simulink model "snb_d"  (R2012b)
settings: Solver=FixedStepDiscrete  SolverMode=SingleTasking  StartTime=0.0  StopTime=10000  RelTol=1e-3
undefined symbols (not defined in the file): Down, pfb_coeff_gen_calc, Up, xlipgetpartsetting
libraries: xbsIndex_r4 x12106, casper_library_misc x14, casper_library_communications x8, casper_library_delays x1, xps_library x1
(part 24 of 79)

== system snb_d/mix_dec_fir/dec_fir_async1 ==
  sync_in : Inport
  dv_in : Inport  Port=2
  dbus_in : Inport  Port=3
  convert1 : xbsIndex_r4/Convert  gui_display_data_type=Fixed-point  arith_type="Signed  (2's comp)"  n_bits=18  bin_pt=17  float_type=Single  exp_bits=8  fraction_bits=24  quantization="Round  (unbiased: +/- Inf)"  overflow=Wrap  en=off  latency=3  dbl_ovrd=off  pipeline=off  block_type=convert
  convert2 : xbsIndex_r4/Convert  gui_display_data_type=Fixed-point  arith_type="Signed  (2's comp)"  n_bits=18  bin_pt=17  float_type=Single  exp_bits=8  fraction_bits=24  quantization="Round  (unbiased: +/- Inf)"  overflow=Wrap  en=off  latency=3  dbl_ovrd=off  pipeline=off  block_type=convert
  dv_delay : xbsIndex_r4/Delay  rst=off  infoeditControl=Selection of Reset will increase slice count due to use of real FFs and instead of SRLs  en=off  latency=18  dbl_ovrd=off  reg_retiming=off  block_type=delay
  fir_col_async1 : Subsystem  AncestorBlock=casper_library_downconverter/fir_col_async  mask(fir_col_async){n_inputs=8, coeff=[0.12401     0.11348    0.094703    0.071556    0.048306    0.028458    0.013979   0.0055083], add_latency=3, mult_latency=3, coeff_bit_width=24, coeff_bin_pt=23, first_stage_hdl=on, adder_imp=DSP48, async=on, bus_input=on, input_width=20, input_bp=18, input_type=Signed, dbl=on}
      mask prompts: n_inputs "Inputs"; coeff "Coefficients"; add_latency "Add latency"; mult_latency "Mult Latency"; coeff_bit_width "Coefficient bit width"; coeff_bin_pt "Coefficient binary point"; first_stage_hdl "Implement first stage of adder trees on output as behavioural HDL"; adder_imp "Adder implementation"; async "Asynchronous ops"; bus_input "Bus input"; input_width "Input bitwidth"; input_bp "Input binary point"; input_type "Input datatype"; dbl "Double col"
      mask init:
      | fir_col_async_init(gcb);
      mask Help: eval('xlWeb(''http://casper.berkeley.edu/wiki/Fir_col'')')
      mask TypeOptions adder_imp: Behavioral | Fabric | DSP48
      mask Callback bus_input:
      | onoff = get_param(gcb, 'bus_input');
      | set_param_state(gcb, 'input_width', onoff)
      | set_param_state(gcb, 'input_bp', onoff)
      | set_param_state(gcb, 'input_type', onoff)
      mask TypeOptions input_type: Signed | Unsigned
  imag_sum : Subsystem  AncestorBlock=casper_library_misc/adder_tree  mask(adder_tree){n_inputs=1, latency=3, adder_imp=DSP48, first_stage_hdl=off}
      mask prompts: n_inputs "Number of Inputs"; latency "Add Latency"; adder_imp "Adder implementation"; first_stage_hdl "Use behavioural HDL for first stage of adders"
      mask help:
      | Sums all inputs using a tree of adds and delays.
      |
      | Number of inputs: The number of inputs to the block to be summed
      | Add latency: The number of clock cycles to perform one addition (affects timing)..
      | Adder implementation: choice of fabric or DSP48E core, or behavioral HDL
      | Use behavioural HDL for first stage of adders: Causes the first stage of adders to be absorbed into DSP blocks if multipliers precede them (Virtex 5). Overrides Adder implementation
      mask init:
      | adder_tree_init(gcb, ...
      |     'n_inputs', n_inputs, ...
      |     'latency', latency, ...
      |     'adder_imp', adder_imp, ...
      |     'first_stage_hdl', first_stage_hdl);
      settings: AttributesFormatString=latency 0
      mask Help: eval('xlWeb(''http://casper.berkeley.edu/wiki/Adder_tree'')')
      mask TypeOptions adder_imp: Behavioral | Fabric | DSP48
  real_sum : Subsystem  AncestorBlock=casper_library_misc/adder_tree  mask(adder_tree){n_inputs=1, latency=3, adder_imp=DSP48, first_stage_hdl=off}
      mask prompts: n_inputs "Number of Inputs"; latency "Add Latency"; adder_imp "Adder implementation"; first_stage_hdl "Use behavioural HDL for first stage of adders"
      mask help:
      | Sums all inputs using a tree of adds and delays.
      |
      | Number of inputs: The number of inputs to the block to be summed
      | Add latency: The number of clock cycles to perform one addition (affects timing)..
      | Adder implementation: choice of fabric or DSP48E core, or behavioral HDL
      | Use behavioural HDL for first stage of adders: Causes the first stage of adders to be absorbed into DSP blocks if multipliers precede them (Virtex 5). Overrides Adder implementation
      mask init:
      | adder_tree_init(gcb, ...
      |     'n_inputs', n_inputs, ...
      |     'latency', latency, ...
      |     'adder_imp', adder_imp, ...
      |     'first_stage_hdl', first_stage_hdl);
      settings: AttributesFormatString=latency 0
      mask Help: eval('xlWeb(''http://casper.berkeley.edu/wiki/Adder_tree'')')
      mask TypeOptions adder_imp: Behavioral | Fabric | DSP48
  ri_to_c : casper_library_misc/ri_to_c
  shift1 : xbsIndex_r4/Shift  shift_dir=Left  shift_bits=0  en=off  latency=0  precision=Full  arith_type="Signed  (2's comp)"  n_bits=16  bin_pt=14  quantization=Truncate  overflow=Wrap  dbl_ovrd=off  block_type=shift
  shift2 : xbsIndex_r4/Shift  shift_dir=Left  shift_bits=0  en=off  latency=0  precision=Full  arith_type="Signed  (2's comp)"  n_bits=16  bin_pt=14  quantization=Truncate  overflow=Wrap  dbl_ovrd=off  block_type=shift
  sync_delay : xbsIndex_r4/Delay  rst=off  infoeditControl=Selection of Reset will increase slice count due to use of real FFs and instead of SRLs  en=off  latency=18  dbl_ovrd=off  reg_retiming=off  block_type=delay
  sync_out : Outport
  dout : Outport  Port=2
  dv_out : Outport  Port=3
  wires:
  sync_in/1 -> sync_delay/1
  dv_in/1 -> dv_delay/1, fir_col_async1/3(dv)
  dv_delay/1 -> dv_out/1
  dbus_in/1 -> fir_col_async1/1(dbus_in)
  fir_col_async1/3(real_sum) -> real_sum/2(din1)
  fir_col_async1/4(imag_sum) -> imag_sum/2(din1)
  real_sum/2(dout) -> shift1/1
  imag_sum/2(dout) -> shift2/1
  shift1/1 -> convert1/1
  shift2/1 -> convert2/1
  convert1/1 -> ri_to_c/1
  convert2/1 -> ri_to_c/2
  ri_to_c/1 -> dout/1
  sync_delay/1 -> real_sum/1(sync), imag_sum/1(sync)
  real_sum/1(sync_out) -> sync_out/1
  fir_col_async1/1(dbus_out) -> fir_col_async1/2(dbus_back_in)

== system snb_d/mix_dec_fir/mixer ==
  sync : Inport
  din1 : Inport  Port=2
  din2 : Inport  Port=3
  din3 : Inport  Port=4
  din4 : Inport  Port=5
  din5 : Inport  Port=6
  din6 : Inport  Port=7
  din7 : Inport  Port=8
  din8 : Inport  Port=9
  dds : Subsystem  AncestorBlock=casper_library_downconverter/dds  mask(dds){freq_div=16, freq=4, num_lo=8, n_bits=10, latency=2}
      mask prompts: freq_div "Frequency divisions (M)"; freq "Frequency (? / M*2pi)"; num_lo "Parallel LOs"; n_bits "Bit Width"
      mask help:
      | Generates P channels of sin and cos data for mixing
      | with input data in a DDC. To generate frequency
      | N/M(Fc x P) (where Fc is the clock rate)
      | M = "Frequency Divisions", N = "Frequency",
      | Parallel LOs = P
      mask init:
      | dds_init(gcb, ...
      |     'freq_div', freq_div, ...
      |     'freq', freq, ...
      |     'num_lo', num_lo, ...
      |     'n_bits', n_bits, ...
      |     'latency', latency);
      settings: AttributesFormatString=lo at -4/16
      mask Help: eval('xlWeb(''http://casper.berkeley.edu/wiki/Dds'')')
  delay : xbsIndex_r4/Delay  rst=off  infoeditControl=Selection of Reset will increase slice count due to use of real FFs and instead of SRLs  en=off  latency=4  dbl_ovrd=off  reg_retiming=off  block_type=delay
  rcmult1 : Subsystem  AncestorBlock=casper_library_downconverter/rcmult  mask(rcmult){latency=4}
      mask prompts: latency "Multiplier latency"
      mask help:
      | Multiplies input data with cos and sin inputs and
      | outputs results on real and imag ports
      | respectively.
      mask init:
      | rcmult_init(gcb, ...
      |     'latency', latency);
      mask Help: eval('xlWeb(''http://casper.berkeley.edu/wiki/Rcmult'')')
  rcmult2 : Subsystem  AncestorBlock=casper_library_downconverter/rcmult  mask(rcmult){latency=4}
      mask prompts: latency "Multiplier latency"
      mask help:
      | Multiplies input data with cos and sin inputs and
      | outputs results on real and imag ports
      | respectively.
      mask init:
      | rcmult_init(gcb, ...
      |     'latency', latency);
      mask Help: eval('xlWeb(''http://casper.berkeley.edu/wiki/Rcmult'')')
  rcmult3 : Subsystem  AncestorBlock=casper_library_downconverter/rcmult  mask(rcmult){latency=4}
      mask prompts: latency "Multiplier latency"
      mask help:
      | Multiplies input data with cos and sin inputs and
      | outputs results on real and imag ports
      | respectively.
      mask init:
      | rcmult_init(gcb, ...
      |     'latency', latency);
      mask Help: eval('xlWeb(''http://casper.berkeley.edu/wiki/Rcmult'')')
  rcmult4 : Subsystem  AncestorBlock=casper_library_downconverter/rcmult  mask(rcmult){latency=4}
      mask prompts: latency "Multiplier latency"
      mask help:
      | Multiplies input data with cos and sin inputs and
      | outputs results on real and imag ports
      | respectively.
      mask init:
      | rcmult_init(gcb, ...
      |     'latency', latency);
      mask Help: eval('xlWeb(''http://casper.berkeley.edu/wiki/Rcmult'')')
  rcmult5 : Subsystem  AncestorBlock=casper_library_downconverter/rcmult  mask(rcmult){latency=4}
      mask prompts: latency "Multiplier latency"
      mask help:
      | Multiplies input data with cos and sin inputs and
      | outputs results on real and imag ports
      | respectively.
      mask init:
      | rcmult_init(gcb, ...
      |     'latency', latency);
      mask Help: eval('xlWeb(''http://casper.berkeley.edu/wiki/Rcmult'')')
  rcmult6 : Subsystem  AncestorBlock=casper_library_downconverter/rcmult  mask(rcmult){latency=4}
      mask prompts: latency "Multiplier latency"
      mask help:
      | Multiplies input data with cos and sin inputs and
      | outputs results on real and imag ports
      | respectively.
      mask init:
      | rcmult_init(gcb, ...
      |     'latency', latency);
      mask Help: eval('xlWeb(''http://casper.berkeley.edu/wiki/Rcmult'')')
  rcmult7 : Subsystem  AncestorBlock=casper_library_downconverter/rcmult  mask(rcmult){latency=4}
      mask prompts: latency "Multiplier latency"
      mask help:
      | Multiplies input data with cos and sin inputs and
      | outputs results on real and imag ports
      | respectively.
      mask init:
      | rcmult_init(gcb, ...
      |     'latency', latency);
      mask Help: eval('xlWeb(''http://casper.berkeley.edu/wiki/Rcmult'')')
  rcmult8 : Subsystem  AncestorBlock=casper_library_downconverter/rcmult  mask(rcmult){latency=4}
      mask prompts: latency "Multiplier latency"
      mask help:
      | Multiplies input data with cos and sin inputs and
      | outputs results on real and imag ports
      | respectively.
      mask init:
      | rcmult_init(gcb, ...
      |     'latency', latency);
      mask Help: eval('xlWeb(''http://casper.berkeley.edu/wiki/Rcmult'')')
  sync_out : Outport
  real1 : Outport  Port=2
  imag1 : Outport  Port=3
  real2 : Outport  Port=4
  imag2 : Outport  Port=5
  real3 : Outport  Port=6
  imag3 : Outport  Port=7
  real4 : Outport  Port=8
  imag4 : Outport  Port=9
  real5 : Outport  Port=10
  imag5 : Outport  Port=11
  real6 : Outport  Port=12
  imag6 : Outport  Port=13
  real7 : Outport  Port=14
  imag7 : Outport  Port=15
  real8 : Outport  Port=16
  imag8 : Outport  Port=17
  wires:
  sync/1 -> delay/1
  delay/1 -> sync_out/1
  din1/1 -> rcmult1/1(d)
  dds/1(sin0) -> rcmult1/2(sin)
  dds/2(cos0) -> rcmult1/3(cos)
  rcmult1/1(real) -> real1/1
  rcmult1/2(imag) -> imag1/1
  din2/1 -> rcmult2/1(d)
  dds/3(sin1) -> rcmult2/2(sin)
  dds/4(cos1) -> rcmult2/3(cos)
  rcmult2/1(real) -> real2/1
  rcmult2/2(imag) -> imag2/1
  din3/1 -> rcmult3/1(d)
  dds/5(sin2) -> rcmult3/2(sin)
  dds/6(cos2) -> rcmult3/3(cos)
  rcmult3/1(real) -> real3/1
  rcmult3/2(imag) -> imag3/1
  din4/1 -> rcmult4/1(d)
  dds/7(sin3) -> rcmult4/2(sin)
  dds/8(cos3) -> rcmult4/3(cos)
  rcmult4/1(real) -> real4/1
  rcmult4/2(imag) -> imag4/1
  din5/1 -> rcmult5/1(d)
  dds/9(sin4) -> rcmult5/2(sin)
  dds/10(cos4) -> rcmult5/3(cos)
  rcmult5/1(real) -> real5/1
  rcmult5/2(imag) -> imag5/1
  din6/1 -> rcmult6/1(d)
  dds/11(sin5) -> rcmult6/2(sin)
  dds/12(cos5) -> rcmult6/3(cos)
  rcmult6/1(real) -> real6/1
  rcmult6/2(imag) -> imag6/1
  din7/1 -> rcmult7/1(d)
  dds/13(sin6) -> rcmult7/2(sin)
  dds/14(cos6) -> rcmult7/3(cos)
  rcmult7/1(real) -> real7/1
  rcmult7/2(imag) -> imag7/1
  din8/1 -> rcmult8/1(d)
  dds/15(sin7) -> rcmult8/2(sin)
  dds/16(cos7) -> rcmult8/3(cos)
  rcmult8/1(real) -> real8/1
  rcmult8/2(imag) -> imag8/1

== system snb_d/mix_dec_fir/mixer1 ==
  sync : Inport
  din1 : Inport  Port=2
  din2 : Inport  Port=3
  din3 : Inport  Port=4
  din4 : Inport  Port=5
  din5 : Inport  Port=6
  din6 : Inport  Port=7
  din7 : Inport  Port=8
  din8 : Inport  Port=9
  dds : Subsystem  AncestorBlock=casper_library_downconverter/dds  mask(dds){freq_div=16, freq=4, num_lo=8, n_bits=10, latency=2}
      mask prompts: freq_div "Frequency divisions (M)"; freq "Frequency (? / M*2pi)"; num_lo "Parallel LOs"; n_bits "Bit Width"
      mask help:
      | Generates P channels of sin and cos data for mixing
      | with input data in a DDC. To generate frequency
      | N/M(Fc x P) (where Fc is the clock rate)
      | M = "Frequency Divisions", N = "Frequency",
      | Parallel LOs = P
      mask init:
      | dds_init(gcb, ...
      |     'freq_div', freq_div, ...
      |     'freq', freq, ...
      |     'num_lo', num_lo, ...
      |     'n_bits', n_bits, ...
      |     'latency', latency);
      settings: AttributesFormatString=lo at -4/16
      mask Help: eval('xlWeb(''http://casper.berkeley.edu/wiki/Dds'')')
  delay : xbsIndex_r4/Delay  rst=off  infoeditControl=Selection of Reset will increase slice count due to use of real FFs and instead of SRLs  en=off  latency=4  dbl_ovrd=off  reg_retiming=off  block_type=delay
  rcmult1 : Subsystem  AncestorBlock=casper_library_downconverter/rcmult  mask(rcmult){latency=4}
      mask prompts: latency "Multiplier latency"
      mask help:
      | Multiplies input data with cos and sin inputs and
      | outputs results on real and imag ports
      | respectively.
      mask init:
      | rcmult_init(gcb, ...
      |     'latency', latency);
      mask Help: eval('xlWeb(''http://casper.berkeley.edu/wiki/Rcmult'')')
  rcmult2 : Subsystem  AncestorBlock=casper_library_downconverter/rcmult  mask(rcmult){latency=4}
      mask prompts: latency "Multiplier latency"
      mask help:
      | Multiplies input data with cos and sin inputs and
      | outputs results on real and imag ports
      | respectively.
      mask init:
      | rcmult_init(gcb, ...
      |     'latency', latency);
      mask Help: eval('xlWeb(''http://casper.berkeley.edu/wiki/Rcmult'')')
  rcmult3 : Subsystem  AncestorBlock=casper_library_downconverter/rcmult  mask(rcmult){latency=4}
      mask prompts: latency "Multiplier latency"
      mask help:
      | Multiplies input data with cos and sin inputs and
      | outputs results on real and imag ports
      | respectively.
      mask init:
      | rcmult_init(gcb, ...
      |     'latency', latency);
      mask Help: eval('xlWeb(''http://casper.berkeley.edu/wiki/Rcmult'')')
  rcmult4 : Subsystem  AncestorBlock=casper_library_downconverter/rcmult  mask(rcmult){latency=4}
      mask prompts: latency "Multiplier latency"
      mask help:
      | Multiplies input data with cos and sin inputs and
      | outputs results on real and imag ports
      | respectively.
      mask init:
      | rcmult_init(gcb, ...
      |     'latency', latency);
      mask Help: eval('xlWeb(''http://casper.berkeley.edu/wiki/Rcmult'')')
  rcmult5 : Subsystem  AncestorBlock=casper_library_downconverter/rcmult  mask(rcmult){latency=4}
      mask prompts: latency "Multiplier latency"
      mask help:
      | Multiplies input data with cos and sin inputs and
      | outputs results on real and imag ports
      | respectively.
      mask init:
      | rcmult_init(gcb, ...
      |     'latency', latency);
      mask Help: eval('xlWeb(''http://casper.berkeley.edu/wiki/Rcmult'')')
  rcmult6 : Subsystem  AncestorBlock=casper_library_downconverter/rcmult  mask(rcmult){latency=4}
      mask prompts: latency "Multiplier latency"
      mask help:
      | Multiplies input data with cos and sin inputs and
      | outputs results on real and imag ports
      | respectively.
      mask init:
      | rcmult_init(gcb, ...
      |     'latency', latency);
      mask Help: eval('xlWeb(''http://casper.berkeley.edu/wiki/Rcmult'')')
  rcmult7 : Subsystem  AncestorBlock=casper_library_downconverter/rcmult  mask(rcmult){latency=4}
      mask prompts: latency "Multiplier latency"
      mask help:
      | Multiplies input data with cos and sin inputs and
      | outputs results on real and imag ports
      | respectively.
      mask init:
      | rcmult_init(gcb, ...
      |     'latency', latency);
      mask Help: eval('xlWeb(''http://casper.berkeley.edu/wiki/Rcmult'')')
  rcmult8 : Subsystem  AncestorBlock=casper_library_downconverter/rcmult  mask(rcmult){latency=4}
      mask prompts: latency "Multiplier latency"
      mask help:
      | Multiplies input data with cos and sin inputs and
      | outputs results on real and imag ports
      | respectively.
      mask init:
      | rcmult_init(gcb, ...
      |     'latency', latency);
      mask Help: eval('xlWeb(''http://casper.berkeley.edu/wiki/Rcmult'')')
  sync_out : Outport
  real1 : Outport  Port=2
  imag1 : Outport  Port=3
  real2 : Outport  Port=4
  imag2 : Outport  Port=5
  real3 : Outport  Port=6
  imag3 : Outport  Port=7
  real4 : Outport  Port=8
  imag4 : Outport  Port=9
  real5 : Outport  Port=10
  imag5 : Outport  Port=11
  real6 : Outport  Port=12
  imag6 : Outport  Port=13
  real7 : Outport  Port=14
  imag7 : Outport  Port=15
  real8 : Outport  Port=16
  imag8 : Outport  Port=17
  wires:
  rcmult8/2(imag) -> imag8/1
  rcmult8/1(real) -> real8/1
  dds/16(cos7) -> rcmult8/3(cos)
  dds/15(sin7) -> rcmult8/2(sin)
  din8/1 -> rcmult8/1(d)
  rcmult7/2(imag) -> imag7/1
  rcmult7/1(real) -> real7/1
  dds/14(cos6) -> rcmult7/3(cos)
  dds/13(sin6) -> rcmult7/2(sin)
  din7/1 -> rcmult7/1(d)
  rcmult6/2(imag) -> imag6/1
  rcmult6/1(real) -> real6/1
  dds/12(cos5) -> rcmult6/3(cos)
  dds/11(sin5) -> rcmult6/2(sin)
  din6/1 -> rcmult6/1(d)
  rcmult5/2(imag) -> imag5/1
  rcmult5/1(real) -> real5/1
  dds/10(cos4) -> rcmult5/3(cos)
  dds/9(sin4) -> rcmult5/2(sin)
  din5/1 -> rcmult5/1(d)
  rcmult4/2(imag) -> imag4/1
  rcmult4/1(real) -> real4/1
  dds/8(cos3) -> rcmult4/3(cos)
  dds/7(sin3) -> rcmult4/2(sin)
  din4/1 -> rcmult4/1(d)
  rcmult3/2(imag) -> imag3/1
  rcmult3/1(real) -> real3/1
  dds/6(cos2) -> rcmult3/3(cos)
  dds/5(sin2) -> rcmult3/2(sin)
  din3/1 -> rcmult3/1(d)
  rcmult2/2(imag) -> imag2/1
  rcmult2/1(real) -> real2/1
  dds/4(cos1) -> rcmult2/3(cos)
  dds/3(sin1) -> rcmult2/2(sin)
  din2/1 -> rcmult2/1(d)
  rcmult1/2(imag) -> imag1/1
  rcmult1/1(real) -> real1/1
  dds/2(cos0) -> rcmult1/3(cos)
  dds/1(sin0) -> rcmult1/2(sin)
  din1/1 -> rcmult1/1(d)
  delay/1 -> sync_out/1
  sync/1 -> delay/1

== system snb_d/mix_dec_fir/pipeline1 ==
  d : Inport
  Register0 : xbsIndex_r4/Register  init=0  rst=off  en=off  dbl_ovrd=off  block_type=register
      settings: block_version=11.4
  q : Outport
  wires:
  d/1 -> Register0/1
  Register0/1 -> q/1

== system snb_d/mix_dec_fir/pipeline2 ==
  d : Inport
  Register0 : xbsIndex_r4/Register  init=0  rst=off  en=off  dbl_ovrd=off  block_type=register
      settings: block_version=11.4
  q : Outport
  wires:
  d/1 -> Register0/1
  Register0/1 -> q/1

== system snb_d/mix_dec_fir/pipeline29 ==
  d : Inport
  Register0 : xbsIndex_r4/Register  init=0  rst=off  en=off  dbl_ovrd=off  block_type=register
      settings: block_version=11.4
  q : Outport
  wires:
  d/1 -> Register0/1
  Register0/1 -> q/1

== system snb_d/mix_dec_fir/pipeline3 ==
  d : Inport
  Register0 : xbsIndex_r4/Register  init=0  rst=off  en=off  dbl_ovrd=off  block_type=register
      settings: block_version=11.4
  q : Outport
  wires:
  d/1 -> Register0/1
  Register0/1 -> q/1

== system snb_d/mix_dec_fir/pipeline4 ==
  d : Inport
  Register0 : xbsIndex_r4/Register  init=0  rst=off  en=off  dbl_ovrd=off  block_type=register
      settings: block_version=11.4
  q : Outport
  wires:
  d/1 -> Register0/1
  Register0/1 -> q/1

== system snb_d/mix_dec_fir/pipeline5 ==
  d : Inport
  Register0 : xbsIndex_r4/Register  init=0  rst=off  en=off  dbl_ovrd=off  block_type=register
      settings: block_version=11.4
  q : Outport
  wires:
  d/1 -> Register0/1
  Register0/1 -> q/1

== system snb_d/oneshot/edge_detect1 ==
  in : Inport
  Delay : xbsIndex_r4/Delay  rst=off  infoeditControl=Selection of Reset will increase slice count due to use of real FFs and instead of SRLs  en=off  latency=1  dbl_ovrd=off  reg_retiming=off  block_type=delay
      settings: xl_area=[0, 0, 0, 0, 0, 0, 0]
  Inverter : xbsIndex_r4/Inverter  en=off  latency=0  dbl_ovrd=off  block_type=inv
      settings: xl_area=[0, 0, 0, 0, 0, 0, 0]
  edge_op : xbsIndex_r4/Logical  logical_function=NOR  inputs=2  en=off  latency=0  precision=Full  arith_type=Unsigned  n_bits=8  bin_pt=2  align_bp=on  dbl_ovrd=off  block_type=logical
      settings: xl_area=[0, 0, 0, 0, 0, 0, 0]
  out : Outport
  wires:
  Delay/1 -> edge_op/2
  in/1 -> Delay/1, Inverter/1
  edge_op/1 -> out/1
  Inverter/1 -> edge_op/1

== system snb_d/oneshot1/edge_detect1 ==
  in : Inport
  Delay : xbsIndex_r4/Delay  rst=off  infoeditControl=Selection of Reset will increase slice count due to use of real FFs and instead of SRLs  en=off  latency=1  dbl_ovrd=off  reg_retiming=off  block_type=delay
      settings: xl_area=[0, 0, 0, 0, 0, 0, 0]
  Inverter : xbsIndex_r4/Inverter  en=off  latency=0  dbl_ovrd=off  block_type=inv
      settings: xl_area=[0, 0, 0, 0, 0, 0, 0]
  edge_op : xbsIndex_r4/Logical  logical_function=NOR  inputs=2  en=off  latency=0  precision=Full  arith_type=Unsigned  n_bits=8  bin_pt=2  align_bp=on  dbl_ovrd=off  block_type=logical
      settings: xl_area=[0, 0, 0, 0, 0, 0, 0]
  out : Outport
  wires:
  Inverter/1 -> edge_op/1
  edge_op/1 -> out/1
  in/1 -> Inverter/1, Delay/1
  Delay/1 -> edge_op/2

== system snb_d/oneshot2/edge_detect1 ==
  in : Inport
  Delay : xbsIndex_r4/Delay  rst=off  infoeditControl=Selection of Reset will increase slice count due to use of real FFs and instead of SRLs  en=off  latency=1  dbl_ovrd=off  reg_retiming=off  block_type=delay
      settings: xl_area=[0, 0, 0, 0, 0, 0, 0]
  Inverter : xbsIndex_r4/Inverter  en=off  latency=0  dbl_ovrd=off  block_type=inv
      settings: xl_area=[0, 0, 0, 0, 0, 0, 0]
  edge_op : xbsIndex_r4/Logical  logical_function=NOR  inputs=2  en=off  latency=0  precision=Full  arith_type=Unsigned  n_bits=8  bin_pt=2  align_bp=on  dbl_ovrd=off  block_type=logical
      settings: xl_area=[0, 0, 0, 0, 0, 0, 0]
  out : Outport
  wires:
  Delay/1 -> edge_op/2
  in/1 -> Delay/1, Inverter/1
  edge_op/1 -> out/1
  Inverter/1 -> edge_op/1

== system snb_d/pack/bus_expand ==
  bus_in : Inport
  reinterpret{1..4} (4 alike) : xbsIndex_r4/Reinterpret  force_arith_type=on  arith_type=Unsigned  force_bin_pt=on  bin_pt=0  block_type=reinterpret
  slice1 : xbsIndex_r4/Slice  nbits=64  boolean_output=off  mode=Upper Bit Location + Width  bit1=-192  base1=MSB of Input  bit0=0  base0=LSB of Input  dbl_ovrd=off  block_type=slice
  slice2 : xbsIndex_r4/Slice  nbits=64  boolean_output=off  mode=Upper Bit Location + Width  bit1=-128  base1=MSB of Input  bit0=0  base0=LSB of Input  dbl_ovrd=off  block_type=slice
  slice3 : xbsIndex_r4/Slice  nbits=64  boolean_output=off  mode=Upper Bit Location + Width  bit1=-64  base1=MSB of Input  bit0=0  base0=LSB of Input  dbl_ovrd=off  block_type=slice
  slice4 : xbsIndex_r4/Slice  nbits=64  boolean_output=off  mode=Upper Bit Location + Width  bit1=0  base1=MSB of Input  bit0=0  base0=LSB of Input  dbl_ovrd=off  block_type=slice
  msb_out4 : Outport
  out3 : Outport  Port=2
  out2 : Outport  Port=3
  lsb_out1 : Outport  Port=4
  wires:
  reinterpret1/1 -> lsb_out1/1
  slice1/1 -> reinterpret1/1
  reinterpret2/1 -> out2/1
  slice2/1 -> reinterpret2/1
  reinterpret3/1 -> out3/1
  slice3/1 -> reinterpret3/1
  reinterpret4/1 -> msb_out4/1
  slice4/1 -> reinterpret4/1
  bus_in/1 -> slice1/1, slice2/1, slice3/1, slice4/1

== system snb_d/pack/bus_expand1 ==
  bus_in : Inport
  reinterpret{1..4} (4 alike) : xbsIndex_r4/Reinterpret  force_arith_type=on  arith_type=Unsigned  force_bin_pt=on  bin_pt=0  block_type=reinterpret
  slice1 : xbsIndex_r4/Slice  nbits=1  boolean_output=off  mode=Upper Bit Location + Width  bit1=-3  base1=MSB of Input  bit0=0  base0=LSB of Input  dbl_ovrd=off  block_type=slice
  slice2 : xbsIndex_r4/Slice  nbits=1  boolean_output=off  mode=Upper Bit Location + Width  bit1=-2  base1=MSB of Input  bit0=0  base0=LSB of Input  dbl_ovrd=off  block_type=slice
  slice3 : xbsIndex_r4/Slice  nbits=1  boolean_output=off  mode=Upper Bit Location + Width  bit1=-1  base1=MSB of Input  bit0=0  base0=LSB of Input  dbl_ovrd=off  block_type=slice
  slice4 : xbsIndex_r4/Slice  nbits=1  boolean_output=off  mode=Upper Bit Location + Width  bit1=0  base1=MSB of Input  bit0=0  base0=LSB of Input  dbl_ovrd=off  block_type=slice
  msb_out4 : Outport
  out3 : Outport  Port=2
  out2 : Outport  Port=3
  lsb_out1 : Outport  Port=4
  wires:
  reinterpret1/1 -> lsb_out1/1
  slice1/1 -> reinterpret1/1
  reinterpret2/1 -> out2/1
  slice2/1 -> reinterpret2/1
  reinterpret3/1 -> out3/1
  slice3/1 -> reinterpret3/1
  reinterpret4/1 -> msb_out4/1
  slice4/1 -> reinterpret4/1
  bus_in/1 -> slice1/1, slice2/1, slice3/1, slice4/1

== system snb_d/pack/bus_expand2 ==
  bus_in : Inport
  reinterpret{1..4} (4 alike) : xbsIndex_r4/Reinterpret  force_arith_type=on  arith_type=Unsigned  force_bin_pt=on  bin_pt=0  block_type=reinterpret
  slice1 : xbsIndex_r4/Slice  nbits=16  boolean_output=off  mode=Upper Bit Location + Width  bit1=-48  base1=MSB of Input  bit0=0  base0=LSB of Input  dbl_ovrd=off  block_type=slice
  slice2 : xbsIndex_r4/Slice  nbits=16  boolean_output=off  mode=Upper Bit Location + Width  bit1=-32  base1=MSB of Input  bit0=0  base0=LSB of Input  dbl_ovrd=off  block_type=slice
  slice3 : xbsIndex_r4/Slice  nbits=16  boolean_output=off  mode=Upper Bit Location + Width  bit1=-16  base1=MSB of Input  bit0=0  base0=LSB of Input  dbl_ovrd=off  block_type=slice
  slice4 : xbsIndex_r4/Slice  nbits=16  boolean_output=off  mode=Upper Bit Location + Width  bit1=0  base1=MSB of Input  bit0=0  base0=LSB of Input  dbl_ovrd=off  block_type=slice
  msb_out4 : Outport
  out3 : Outport  Port=2
  out2 : Outport  Port=3
  lsb_out1 : Outport  Port=4
  wires:
  bus_in/1 -> slice4/1, slice3/1, slice2/1, slice1/1
  slice4/1 -> reinterpret4/1
  reinterpret4/1 -> msb_out4/1
  slice3/1 -> reinterpret3/1
  reinterpret3/1 -> out3/1
  slice2/1 -> reinterpret2/1
  reinterpret2/1 -> out2/1
  slice1/1 -> reinterpret1/1
  reinterpret1/1 -> lsb_out1/1

== system snb_d/pack/pipeline1 ==
  d : Inport
  Register0 : xbsIndex_r4/Register  init=0  rst=off  en=off  dbl_ovrd=off  block_type=register
      settings: block_version=11.4
  Register1 : xbsIndex_r4/Register  init=0  rst=off  en=off  dbl_ovrd=off  block_type=register
      settings: block_version=11.4
  q : Outport
  wires:
  Register1/1 -> q/1
  d/1 -> Register0/1
  Register0/1 -> Register1/1

== system snb_d/pack/pipeline2 ==
  d : Inport
  Register0 : xbsIndex_r4/Register  init=0  rst=off  en=off  dbl_ovrd=off  block_type=register
      settings: block_version=11.4
  q : Outport
  wires:
  d/1 -> Register0/1
  Register0/1 -> q/1

== system snb_d/pack/pipeline3 ==
  d : Inport
  Register0 : xbsIndex_r4/Register  init=0  rst=off  en=off  dbl_ovrd=off  block_type=register
      settings: block_version=11.4
  Register1 : xbsIndex_r4/Register  init=0  rst=off  en=off  dbl_ovrd=off  block_type=register
      settings: block_version=11.4
  q : Outport
  wires:
  Register1/1 -> q/1
  d/1 -> Register0/1
  Register0/1 -> Register1/1

== system snb_d/pack/pipeline4 ==
  d : Inport
  Register0 : xbsIndex_r4/Register  init=0  rst=off  en=off  dbl_ovrd=off  block_type=register
      settings: block_version=11.4
  Register1 : xbsIndex_r4/Register  init=0  rst=off  en=off  dbl_ovrd=off  block_type=register
      settings: block_version=11.4
  q : Outport
  wires:
  Register0/1 -> Register1/1
  d/1 -> Register0/1
  Register1/1 -> q/1

== system snb_d/pack/pipeline5 ==
  d : Inport
  Register0 : xbsIndex_r4/Register  init=0  rst=off  en=off  dbl_ovrd=off  block_type=register
      settings: block_version=11.4
  Register1 : xbsIndex_r4/Register  init=0  rst=off  en=off  dbl_ovrd=off  block_type=register
      settings: block_version=11.4
  q : Outport
  wires:
  Register1/1 -> q/1
  d/1 -> Register0/1
  Register0/1 -> Register1/1

== system snb_d/pack/pipeline50 ==
  d : Inport
  Register0 : xbsIndex_r4/Register  init=0  rst=off  en=off  dbl_ovrd=off  block_type=register
      settings: block_version=11.4
  Register1 : xbsIndex_r4/Register  init=0  rst=off  en=off  dbl_ovrd=off  block_type=register
      settings: block_version=11.4
  q : Outport
  wires:
  Register0/1 -> Register1/1
  d/1 -> Register0/1
  Register1/1 -> q/1

== system snb_d/pack/pipeline6 ==
  d : Inport
  Register0 : xbsIndex_r4/Register  init=0  rst=off  en=off  dbl_ovrd=off  block_type=register
      settings: block_version=11.4
  Register1 : xbsIndex_r4/Register  init=0  rst=off  en=off  dbl_ovrd=off  block_type=register
      settings: block_version=11.4
  q : Outport
  wires:
  Register0/1 -> Register1/1
  d/1 -> Register0/1
  Register1/1 -> q/1

== system snb_d/pack/pipeline7 ==
  d : Inport
  Register0 : xbsIndex_r4/Register  init=0  rst=off  en=off  dbl_ovrd=off  block_type=register
      settings: block_version=11.4
  Register1 : xbsIndex_r4/Register  init=0  rst=off  en=off  dbl_ovrd=off  block_type=register
      settings: block_version=11.4
  q : Outport
  wires:
  Register1/1 -> q/1
  d/1 -> Register0/1
  Register0/1 -> Register1/1
